simulink library "sps_library"  (R2025a)
settings: Solver=VariableStepAuto  StartTime=0.0  StopTime=10.0  RelTol=1e-3
undefined symbols (not defined in the file): bus, c_dc, gfli_b, inf_src, line_ns, ts
libraries: spsBreakerLib x7, spsabctodq0Lib x6, spsThreePhaseVIMeasurementLib x4, spsThreePhaseParallelRLCLoadLib x4, spsSeriesRLCBranchLib x3, spsThreePhaseSeriesRLCBranchLib x3, spsControlledCurrentSourceLib x2, spsDCVoltageSourceLib x2, spsGroundLib x2, spsThreePhaseBreakerLib x2, spsThreePhaseSourceLib x2, spsRMSLib x1
settings Model: Creator=paul  LastModifiedBy=paul

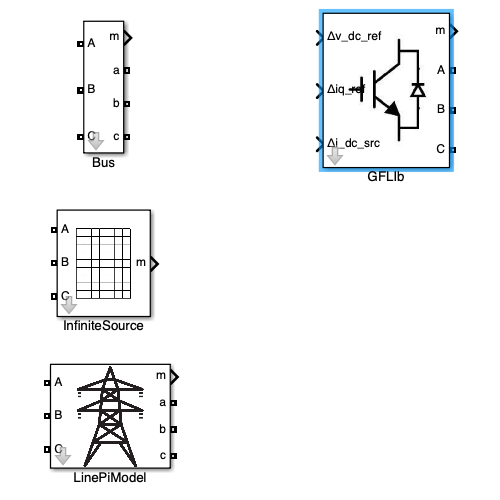
[thumbnail: Simulink's stored preview of the top-level diagram]
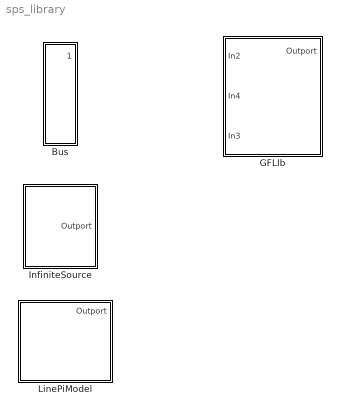
== system sps_library ==
  Bus : Subsystem  mask{s=bus{1}, sbase=100000000, vbase=230000, fbase=60}
      mask prompts: s "Structure from Workspace"; sbase "Sbase (3-phase VA)"; vbase "Vbase (L-L Vrms)"; fbase "Frequency (Hz)"
      mask init:
      | % Get simulink block as class. "m" is now a class
      | m = Simulink.Mask.get(gcb);
      | 
      | % Get an array of all parameters of the column "Name" of "Parameters & Dialog" tab
      | % For example, all_parameters = ['sbase', 'vbase']
      | all_parameters = m.Parameters;
      | 
      | % Iterate over all parameters and assign the field values of the structure
      | % in the workspace to the parameters of the current simulink block.
      | % The variable "st" must be defined in "Parameters & Dialog". 
      | 
      | for i = 1:numel(all_parameters)
      |     param_name = all_parameters(i).Name; % get parameter name of the simulink block
      |     if isfield(s, param_name) % check if field exist in the structure
      |         new_value = string(getfield(s, param_name)); % get the value of the structure field
      |         set_param(gcb, param_name, new_value); % assign the value of structure to simulink block
      |     end
      | end
      mask DialogControl DescGroupVar Prompt: Bus and measurements
      mask DialogControl Bus Prompt: Measure voltage, magnitude and phase, active power, reactive power. Note: Default current flow direction goes from uppercase (ABC) to lowercase (abc). Author: STING developers.
      mask DialogControl Container2 Prompt: Parameters
      mask DialogControl Control2 Prompt: Enter below the structure defined in your current Matlab workspace that contains parameters, power flow solution, initial conditions, etc. Click on "Apply" to migrate data to this block.
  GFLIb : Subsystem  mask{s=gfli_b{1}}
      mask prompts: s "Structure from workspace"
      mask init:
      | m = Simulink.Mask.get(gcb);
      |  
      | % Get all major boxes, like parameters, emt initial conditions
      | all_diagcontrols = m.getDialogControls();
      | 
      | for i=1:length(all_diagcontrols)
      | 
      |     control = all_diagcontrols(i);  
      |     control_name = control.Name; % name of box, for example: parameters, emt_init_cond
      |     control_fields = control.DialogControls; % all sub-boxes, like [sbase, vbase]
      | 
      |     for j=1:length(control_fields)
      | 
      |         param_name = control_fields(j).Name; % for example: sbase
      | 
      |         if isfield(s, param_name) % check if field exist in the structure
      |             new_value = string(getfield(s, param_name)); % get the value of the structure field
      |             set_param(gcb, param_name, new_value); % assign the value of structure to simulink block
      |         
      |         elseif isfield(s,control_name) % check if there is a structure inside of the structure
      |             x = getfield(s, control_name);
      |             if isfield(x, param_name)
      |                 new_value = string(getfield(x, param_name)); 
      |                 set_param(gcb, param_name, new_value);
      |             end
      | 
      |         end
      | 
      |     end
      | 
      | end
      mask DialogControl DescGroupVar Prompt: GFLIb
      mask DialogControl DescTextVar Prompt: Implements the GFLIb class from STING. It is a GFLI that includes PLL, L filter, current controller, and DC-side voltage controller. Author: STING developers.
      mask DialogControl Control2 Prompt: Enter below the structure defined in your current Matlab workspace that contains parameters, power flow solution, initial conditions, etc. Click on "Apply" to migrate data to this block.
      mask Display: image('IBR.jpeg');
  InfiniteSource : Subsystem  mask{s=inf_src{1}}
      mask prompts: s "Structure from workspace"
      mask init:
      | m = Simulink.Mask.get(gcb);
      | 
      | % Get all major boxes, like parameters, emt initial conditions
      | all_diagcontrols = m.getDialogControls();
      | 
      | for i=1:length(all_diagcontrols)
      | 
      |     control = all_diagcontrols(i);  
      |     control_name = control.Name; % name of box, for example: parameters, emt_init_cond
      |     control_fields = control.DialogControls; % all sub-boxes, like [sbase, vbase]
      | 
      |     for j=1:length(control_fields)
      | 
      |         param_name = control_fields(j).Name; % for example: sbase
      | 
      |         if isfield(s, param_name) % check if field exist in the structure
      |             new_value = string(getfield(s, param_name)); % get the value of the structure field
      |             set_param(gcb, param_name, new_value); % assign the value of structure to simulink block
      |         
      |         elseif isfield(s,control_name) % check if there is a structure inside of the structure
      |             x = getfield(s, control_name);
      |             new_value = string(getfield(x, param_name)); 
      |             set_param(gcb, param_name, new_value);
      | 
      |         end
      | 
      |     end
      | 
      | end
      mask DialogControl DescGroupVar Prompt: Infinite Source
      mask DialogControl DescTextVar Prompt: Implements the class InfiniteSource from STING. Author: STING developers.
      mask DialogControl Container2 Prompt: Parameters
      mask DialogControl Control2 Prompt: Enter below the structure defined in your current Matlab workspace that contains parameters, power flow solution, initial conditions, etc. Click on "Apply" to migrate data to this block.
      mask Display: image('grid.jpg', [0,0,0,0,80,80]);
  LinePiModel : Subsystem  mask{s=line_ns{1}}
      mask prompts: s "Structure from workspace"
      mask DialogControl DescGroupVar Prompt: Pi-model of transmission line
      mask DialogControl DescTextVar Prompt: Implements the class LinePiModel from STING. It is a transmission line that includes two shunt impendances and one series impendance. Author: STING developers.
      mask DialogControl Container2 Prompt: Parameters
      mask DialogControl Control2 Prompt: Enter below the structure defined in your current Matlab workspace that contains parameters, power flow solution, initial conditions, etc. Click on "Apply" to migrate data to this block.
      mask Display: image('tx_wo_se.jpg', [0,0,0,0,70,100]);

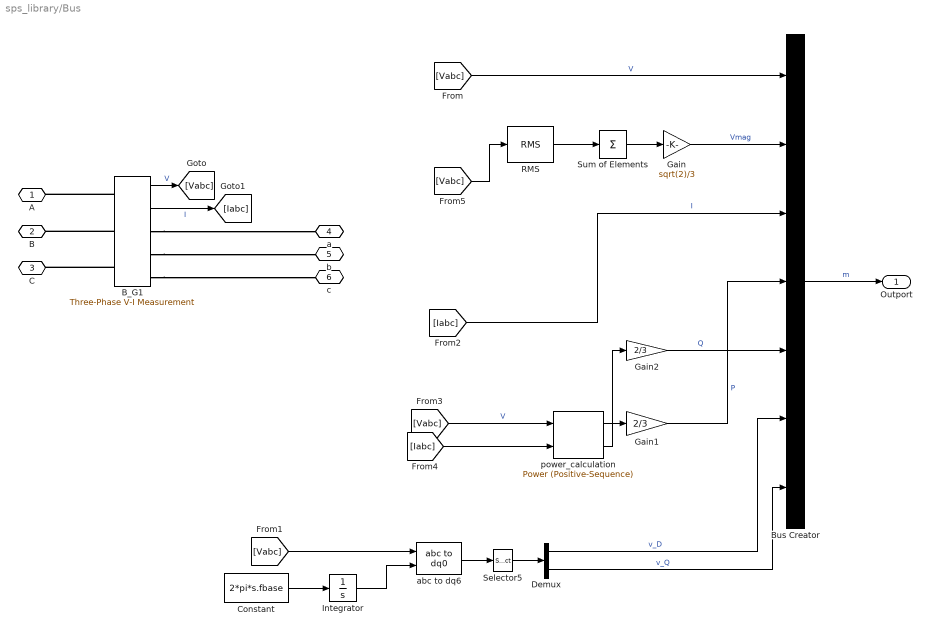
== system sps_library/Bus ==
  B_G1 : spsThreePhaseVIMeasurementLib/Three-Phase V-I Measurement  VoltageMeasurement=phase-to-ground  SetLabelV=off  LabelV=G1_Vabc  Vpu=on  VpuLL=off  CurrentMeasurement=yes  SetLabelI=off  LabelI=G1_Iabc  Ipu=on  Pbase=sbase  Vbase=vbase  OutputType=Complex  PhasorSimulation=off  PSBequivalent=0
  Bus Creator : BusCreator  Inputs=7
  Constant : Constant  Value=2*pi*s.fbase
  Demux : Demux  Outputs=2
  Gain : Gain  Gain=sqrt(2)/3
  Gain1 : Gain  Gain=2/3
  Gain2 : Gain  Gain=2/3
  Integrator : Integrator
  RMS : spsRMSLib/RMS  TrueRMS=on  Freq=fbase  RMSInit=1/sqrt(2)  Ts=0
  Selector5 : Selector  InputPortWidth=3  IndexOptions=Index vector (dialog)  Indices=[1 2]  OutputSizes=1
  Sum of Elements : Sum  Inputs=+
  abc to dq6 : spsabctodq0Lib/abc to dq0  Alignment=Aligned with phase A axis
  power_calculation : spsPowerPositiveSequenceLib/Power (Positive-Sequence)  Freq=fbase  Vinit=[1, 0]  Iinit=[0, 0]  Ts=ts
  A : PMIOPort  Side=Left
  B : PMIOPort  Port=2  Side=Left
  C : PMIOPort  Port=3  Side=Left
  a : PMIOPort  Port=4  Side=Right
  b : PMIOPort  Port=5  Side=Right
  c : PMIOPort  Port=6  Side=Right
  Outport : Outport
  wires:
  Bus Creator/1 -> Outport/1  "m"
  Gain1/1 -> Bus Creator/4  "P"
  Gain2/1 -> Bus Creator/5  "Q"
  B_G1/1 -> [Vabc]  "V"
  [Vabc] -> Bus Creator/1  "V"
  B_G1/2 -> [Iabc]  "I"
  [Iabc] -> Bus Creator/3  "I"
  [Vabc] -> power_calculation/1  "V"
  [Vabc] -> RMS/1
  RMS/1 -> Sum of Elements/1
  Sum of Elements/1 -> Gain/1
  Gain/1 -> Bus Creator/2  "Vmag"
  power_calculation/1 -> Gain1/1
  [Iabc] -> power_calculation/2
  power_calculation/2 -> Gain2/1
  [Vabc] -> abc to dq6/1
  Demux/2 -> Bus Creator/7  "v_Q"
  Integrator/1 -> abc to dq6/2
  Selector5/1 -> Demux/1
  Constant/1 -> Integrator/1
  Demux/1 -> Bus Creator/6  "v_D"
  abc to dq6/1 -> Selector5/1
  connections:
  B_G1/LConn1 -- A/RConn1
  B_G1/LConn3 -- C/RConn1
  B_G1/RConn2 -- b/RConn1
  B_G1/RConn1 -- a/RConn1
  B_G1/LConn2 -- B/RConn1
  B_G1/RConn3 -- c/RConn1

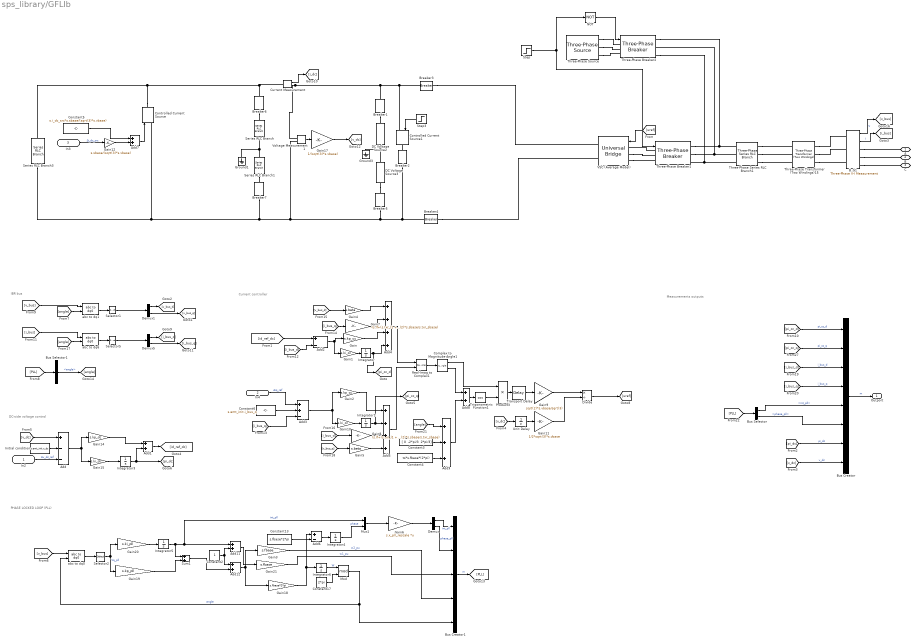
== system sps_library/GFLIb ==
  note: IBR bus
  note: Current controller
  note: Measurements outputs
  note: PHASE LOCKED LOOP (PLL)
  note: DC-side voltage control
  In2 : Inport
  In4 : Inport  Port=2
  In3 : Inport  Port=3
  Add : Sum  Inputs=+--
  Add{1,7..8,11..12} (5 alike) : Sum
  Add2 : Sum  Inputs=+-
  Add3 : Sum  Inputs=++-
  Add4 : Sum  Inputs=++++
  Add5 : Sum  Inputs=++++
  Add6 : Sum  Inputs=+-
  Add9 : Sum  Inputs=+++
  B_G1 : spsThreePhaseVIMeasurementLib/Three-Phase V-I Measurement  VoltageMeasurement=phase-to-ground  SetLabelV=off  LabelV=G1_Vabc  Vpu=on  VpuLL=off  CurrentMeasurement=yes  SetLabelI=off  LabelI=G1_Iabc  Ipu=on  Pbase=s.sbase  Vbase=230*10^3  OutputType=Complex  PhasorSimulation=off  PSBequivalent=0
  Breaker1 : spsBreakerLib/Breaker  InitialState=1  SwitchingTimes=[ts]  External=off  BreakerResistance=1e-7  SnubberResistance=1e6  SnubberCapacitance=inf  Measurements=None  MoreParameters=on  NoBreakLoop=off
  Breaker2 : spsBreakerLib/Breaker  InitialState=1  SwitchingTimes=[ts]  External=off  BreakerResistance=1e-7  SnubberResistance=1e6  SnubberCapacitance=inf  Measurements=None  MoreParameters=on  NoBreakLoop=off
  Breaker{3..4,6..7} (4 alike) : spsBreakerLib/Breaker  InitialState=0  SwitchingTimes=[ts]  External=off  BreakerResistance=1e-7  SnubberResistance=1e6  SnubberCapacitance=inf  Measurements=None  MoreParameters=on  NoBreakLoop=off
  Breaker5 : spsBreakerLib/Breaker  InitialState=1  SwitchingTimes=[ts]  External=off  BreakerResistance=1e-7  SnubberResistance=1e6  SnubberCapacitance=inf  Measurements=None  MoreParameters=on  NoBreakLoop=off
  Bus Creator : BusCreator  Inputs=8
  Bus Creator1 : BusCreator  Inputs=5
  Bus Selector : BusSelector  OutputSignals=int_pll,phase_pll
  Bus Selector1 : BusSelector  OutputSignals=angle
  Complex to Magnitude-Angle1 : ComplexToMagnitudeAngle
  Constant13 : Constant  Value=s.fbase*2*pi
  Constant17 : Constant  Value=2*pi
  Constant2 : Constant
  Constant3 : Constant  Value="[ 0  -2*pi/3  2*pi/3]"
  Constant4 : Constant  Value=ts*s.fbase*(2*pi)
  Constant5 : Constant  Value=s.i_dc_src*s.sbase/(sqrt(3)*s.vbase)
  Constant6 : Constant  Value=s.emt_init.i_bus_q
  Controlled Current Source : spsControlledCurrentSourceLib/Controlled Current Source  Initialize=off  Source_Type=AC  Amplitude=0  Phase=0  Frequency=0  Measurements=None
  Controlled Current Source1 : spsControlledCurrentSourceLib/Controlled Current Source  Initialize=off  Source_Type=AC  Amplitude=0  Phase=0  Frequency=0  Measurements=None
  Current Measurement : spsCurrentMeasurementLib/Current Measurement  PhasorSimulation=off  OutputType=Complex  PSBequivalent=0
  DC Voltage Source2 : spsDCVoltageSourceLib/DC Voltage Source  Amplitude=+sqrt(3)*s.vbase*s.emt_init.v_dc/2  Measurements=None
  DC Voltage Source3 : spsDCVoltageSourceLib/DC Voltage Source  Amplitude=+sqrt(3)*s.vbase*s.emt_init.v_dc/2  Measurements=None
  Demux : Demux  Outputs=2
  Demux1 : Demux  Outputs=2
  Demux5 : Demux  Outputs=2
  Divide : Product  Inputs=*/
  Gain : Gain  Gain=s.kp_cc
  Gain1 : Gain  Gain=s.ki_cc
  Gain10 : Gain  Gain=s.ki_cc
  Gain11 : Gain  Gain=1/2*sqrt(3)*s.vbase
  Gain12 : Gain  Gain=s.sbase/(sqrt(3)*s.vbase)
  Gain14 : Gain  Gain=s.kp_dc
  Gain15 : Gain  Gain=s.ki_dc
  Gain17 : Gain  Gain=1/(sqrt(3)*s.vbase)
  Gain18 : Gain  Gain=s.fbase*2*pi
  Gain19 : Gain  Gain=s.kp_pll
  Gain2 : Gain  Gain=s.kp_cc
  Gain20 : Gain  Gain=s.ki_pll
  Gain21 : Gain  Gain=s.fbase
  Gain3 : Gain  Gain=s.fbase
  Gain4 : Gain  Gain=s.beta
  Gain5 : Gain  Gain=s.beta
  Gain6 : Gain  Gain=s.x_pll_rescale  Multiplication=Matrix(K*u)
  Gain7 : Gain  Gain=-(s.lf+(s.txr_l1 + s.txr_l2)*s.sbase/s.txr_sbase)
  Gain8 : Gain  Gain=(s.lf+(s.txr_l1 + s.txr_l2)*s.sbase/s.txr_sbase)
  Gain9 : Gain  Gain=sqrt(2)*s.vbase/sqrt(3)
  Ground1 : spsGroundLib/Ground  LConnTagsString=a
  Ground3 : spsGroundLib/Ground  LConnTagsString=a
  Initial condition : Constant  Value=s.emt_init.v_dc
  Integrator : Integrator  InitialCondition=s.emt_init.pi_cc_d
  Integrator1 : Integrator  InitialCondition=s.emt_init.pi_cc_q
  Integrator3 : Integrator  InitialCondition=s.emt_init.i_bus_d
  Integrator4 : Integrator  InitialCondition=s.emt_init.angle_ref*pi/180
  Integrator5 : Integrator
  Integrator6 : Integrator  InitialCondition=s.emt_init.angle_ref*pi/180
  Mod : Math  Operator=mod
  Mux1 : Mux  Inputs=2
  NOT : Logic  Operator=NOT  IconShape=distinctive  AllPortsSameDT=off  OutDataTypeStr=boolean
  Product3 : Product  Inputs=**  RndMeth=Zero
  Real-Imag to Complex1 : RealImagToComplex
  Selector1 : Selector  InputPortWidth=3  IndexOptions=Index vector (dialog)  Indices=[1 2]  OutputSizes=1
  Selector2 : Selector  InputPortWidth=3  IndexOptions=Index vector (dialog)  Indices=2  OutputSizes=1
  Selector5 : Selector  InputPortWidth=3  IndexOptions=Index vector (dialog)  Indices=[1 2]  OutputSizes=1
  Series RLC Branch : spsSeriesRLCBranchLib/Series RLC Branch  LConnTagsString=__new0  RConnTagsString=__new0  BranchType=C  Resistance=1  Inductance=1e-3  SetiL0=off  InitialCurrent=0  Capacitance=s.c_dc*1/(3*s.vbase^2/s.sbase)*1/(2*pi*s.fbase)  Setx0=on  InitialVoltage=+sqrt(3)*s.vbase*s.emt_init.v_dc/2  Measurements=None
  Series RLC Branch1 : spsSeriesRLCBranchLib/Series RLC Branch  LConnTagsString=__new0  RConnTagsString=__new0  BranchType=C  Resistance=1  Inductance=1e-3  SetiL0=off  InitialCurrent=0  Capacitance=s.c_dc*1/(3*s.vbase^2/s.sbase)*1/(2*pi*s.fbase)  Setx0=on  InitialVoltage=+sqrt(3)*s.vbase*s.emt_init.v_dc/2  Measurements=None
  Series RLC Branch3 : spsSeriesRLCBranchLib/Series RLC Branch  LConnTagsString=__new0  RConnTagsString=__new0  BranchType=R  Resistance=s.r_dc*(3*s.vbase^2/s.sbase)  Inductance=1e-3  SetiL0=off  InitialCurrent=0  Capacitance=c_dc  Setx0=off  InitialVoltage=0  Measurements=None
  Step : Step  Time=ts  SampleTime=0
  Step3 : Step  Time=ts  Before=s.emt_init.i_out*s.sbase/(sqrt(3)*s.vbase)  After=0  SampleTime=ts
  Sum1 : Sum  SaturateOnIntegerOverflow=on
  Three-Phase Series RLC Branch1 : spsThreePhaseSeriesRLCBranchLib/Three-Phase Series RLC Branch  LConnTagsString=A|B|C  RConnTagsString=A|B|C  BranchType=RL  Resistance=s.rf * s.vbase^2/s.sbase  Inductance=s.lf * s.vbase^2/s.sbase * 1/(2*pi*s.fbase)  Capacitance=1e-6  Measurements=None
  Three-Phase Transformer (Two Windings)15 : spsThreePhaseTransformerTwoWindingsLib/Three-Phase Transformer (Two Windings)  Winding1Connection=Yg  Winding2Connection=Yg  CoreType=Three single-phase transformers  SetSaturation=off  Hysteresis=off  DataFile='hysteresis'  SetInitialFlux=off  Measurements=None  UNITS=pu  NominalPower=[s.txr_sbase , s.fbase ]  Winding1=[ s.vbase , s.txr_r1 , s.txr_l1 ]  Winding2=[ 230*10^3 , s.txr_r2 , s.txr_l2 ]  Rm=1000  Lm=inf  L0=2.866  Saturation=[ 0,0 ; 0.0024,1.2 ; 1.0,1.52 ]  InitialFluxes=[1273.5 -1273.5 1114.3]  BreakLoop=off  DiscreteSolver=Trapezoidal robust  DataType=off  TransfoNumber=1
  Three-Phase Breaker1 : spsThreePhaseBreakerLib/Three-Phase Breaker  InitialState=open  SwitchA=on  SwitchB=on  SwitchC=on  SwitchTimes="[1/60  5/60]"  External=on  BreakerResistance=1e-7  SnubberResistance=1e6  SnubberCapacitance=inf  Measurements=None
  Three-Phase Breaker2 : spsThreePhaseBreakerLib/Three-Phase Breaker  InitialState=closed  SwitchA=on  SwitchB=on  SwitchC=on  SwitchTimes="[1/60  5/60]"  External=on  BreakerResistance=1e-7  SnubberResistance=1e6  SnubberCapacitance=inf  Measurements=None
  Three-Phase Source : spsThreePhaseSourceLib/Three-Phase Source  InternalConnection=Yg  VoltagePhases=off  Voltage=s.emt_init.v_vsc_mag*s.vbase  PhaseAngle=90+s.emt_init.v_vsc_DQ_phase  Voltage_phases=[25e3 25e3 25e3]/sqrt(3)  PhaseAngles_phases=[0 -120 +120]  Frequency=s.fbase  NonIdealSource=off  SpecifyImpedance=off  Resistance=0.8929  Inductance=16.58e-3  ShortCircuitLevel=100e6  BaseVoltage=25e3  XRratio=7  BusType=swing  Pref=10e3  Qref=0  Prefabc=[10e3, 10e3, 10e3]  Qrefabc=[0, 0, 0]  Qmin=-inf  Qmax=inf
  Transport Delay : TransportDelay  DelayTime=ts  InitialOutput=s.emt_init.v_vsc_mag*[cosd(s.emt_init.v_vsc_DQ_phase) cosd(s.emt_init.v_vsc_DQ_phase-120) cosd(s.emt_init.v_vsc_DQ_phase+120)]
  Trigonometric Function1 : Trigonometry  Operator=cos
  Unit Delay : UnitDelay  InitialCondition=s.emt_init.v_dc  SampleTime=ts  HasFrameUpgradeWarning=on
  VSC (Average Model) : spsUniversalBridgeLib/Universal Bridge  Arms=3  SnubberResistance=1e5  SnubberCapacitance=inf  Device=Average-model based VSC  Ron=1e-3  Lon=0  ForwardVoltages="[  0  0  ]"  ForwardVoltage=0  GTOparameters=[ 10e-6 , 20e-6 ]  IGBTparameters=[ 1e-6 , 2e-6 ]  Measurements=None  Measurements_2=None  converterType=Rectifier
  Voltage Measurement1 : spsVoltageMeasurementLib/Voltage Measurement  PhasorSimulation=off  OutputType=Complex  PSBequivalent=0
  abc to dq0 : spsabctodq0Lib/abc to dq0  Alignment=Aligned with phase A axis
  abc to dq1 : spsabctodq0Lib/abc to dq0  Alignment=Aligned with phase A axis
  abc to dq6 : spsabctodq0Lib/abc to dq0  Alignment=Aligned with phase A axis
  A : PMIOPort  Side=Right
  B : PMIOPort  Port=2  Side=Right
  C : PMIOPort  Port=3  Side=Right
  Outport : Outport
  wires:
  Add8/1 -> Trigonometric Function1/1
  [uref] -> VSC (Average Model)/1
  Add5/1 -> Real-Imag to Complex1/2
  Constant3/1 -> Add9/2
  Gain7/1 -> Add4/2
  Gain9/1 -> Divide/1
  Trigonometric Function1/1 -> Product3/2
  [angle] -> Add9/1
  Complex to Magnitude-Angle1/2 -> Add8/1
  Add2/1 -> Gain1/1, Gain/1
  Demux5/2 -> [i_bus_q]
  [angle] -> abc to dq6/2
  Gain4/1 -> Add4/1
  [v_bus_q] -> Gain5/1
  Product3/1 -> Transport Delay/1
  [i_bus] -> abc to dq6/1
  [v_bus_d] -> Gain4/1
  Add4/1 -> Real-Imag to Complex1/1
  Real-Imag to Complex1/1 -> Complex to Magnitude-Angle1/1
  [i_bus_q] -> Gain7/1
  Complex to Magnitude-Angle1/1 -> Product3/1
  abc to dq6/1 -> Selector5/1
  Add9/1 -> Add8/2
  Constant4/1 -> Add9/3
  [i_bus_d] -> Gain8/1
  Gain/1 -> Add4/3
  Demux5/1 -> [i_bus_d]
  Integrator/1 -> Add4/4, [pi_cc_d]
  Gain5/1 -> Add5/4
  Gain8/1 -> Add5/3
  Gain2/1 -> Add5/1
  Add3/1 -> Gain10/1, Gain2/1
  abc to dq1/1 -> Selector1/1
  Demux1/1 -> [v_bus_d]
  Demux1/2 -> [v_bus_q]
  [v_bus] -> abc to dq1/1
  [angle] -> abc to dq1/2
  Gain1/1 -> Integrator/1
  Integrator1/1 -> [pi_cc_q], Add5/2
  Gain10/1 -> Integrator1/1
  Selector1/1 -> Demux1/1
  Selector5/1 -> Demux5/1
  NOT/1 -> Three-Phase Breaker2/1
  Step/1 -> NOT/1, Three-Phase Breaker1/1
  Transport Delay/1 -> Gain9/1
  In4/1 -> Add3/1  "Δiq_ref"
  [pi_cc_d] -> Bus Creator/1  "pi_cc_d"
  [pi_cc_q] -> Bus Creator/2  "pi_cc_q"
  Bus Creator/1 -> Outport/1  "m"
  [i_bus_d] -> Bus Creator/3  "i_bus_d"
  [i_bus_q] -> Bus Creator/4  "i_bus_q"
  [v_dc] -> Unit Delay/1
  Gain11/1 -> Divide/2
  Divide/1 -> [uref]
  B_G1/1 -> [v_bus]  "V"
  B_G1/2 -> [i_bus]  "I"
  [i_bus_q] -> Add3/3
  Constant6/1 -> Add3/2
  Unit Delay/1 -> Gain11/1
  [i_bus_d] -> Add2/2
  In3/1 -> Gain12/1  "Δi_dc_src"
  Voltage Measurement1/1 -> Gain17/1
  Current Measurement/1 -> [i_dc]
  Step3/1 -> Controlled Current Source1/1
  Add7/1 -> Controlled Current Source/1
  Gain17/1 -> [v_dc]
  Constant5/1 -> Add7/1
  Integrator3/1 -> [pi_dc], Add1/2
  Add1/1 -> [id_ref_dc]
  Gain15/1 -> Integrator3/1
  [v_dc] -> Add/1
  Initial condition/1 -> Add/2
  Add/1 -> Gain15/1, Gain14/1
  In2/1 -> Add/3  "Δv_dc_ref"
  Gain14/1 -> Add1/1
  [pi_dc] -> Bus Creator/7  "pi_dc"
  [v_dc] -> Bus Creator/8  "v_dc"
  [id_ref_dc] -> Add2/1
  Constant13/1 -> Add6/2
  Selector2/1 -> Gain20/1, Gain19/1  "Vq_pll"
  Constant17/1 -> Mod/2
  Bus Creator1/1 -> [PLL]  "m"
  Constant2/1 -> Add12/1, Add11/2
  Integrator4/1 -> Mux1/2  "phase"
  Add11/1 -> Gain21/1
  Add12/1 -> Gain18/1, Gain3/1
  Integrator6/1 -> Mod/1  "W"
  Mod/1 -> abc to dq0/2, Bus Creator1/5  "angle"
  Gain18/1 -> Integrator6/1, Add6/1
  Gain20/1 -> Integrator5/1
  Gain3/1 -> Bus Creator1/4  "w2_pu"
  [v_bus] -> abc to dq0/1
  Sum1/1 -> Add12/2
  abc to dq0/1 -> Selector2/1
  Gain19/1 -> Sum1/2
  Add6/1 -> Integrator4/1
  Gain21/1 -> Bus Creator1/3  "w1_pu"
  Bus Selector1/1 -> [angle]  "<angle>"
  [PLL] -> Bus Selector1/1
  [PLL] -> Bus Selector/1
  Integrator5/1 -> Mux1/1, Add11/1, Sum1/1  "int_pll"
  Bus Selector/1 -> Bus Creator/5  "<int_pll>"
  Bus Selector/2 -> Bus Creator/6  "<phase_pll>"
  Mux1/1 -> Gain6/1
  Gain6/1 -> Demux/1
  Demux/1 -> Bus Creator1/1  "int_pll"
  Demux/2 -> Bus Creator1/2  "phase_pll"
  Gain12/1 -> Add7/2
  connections:
  Three-Phase Source/RConn3 -- Three-Phase Breaker2/LConn3
  Three-Phase Source/RConn2 -- Three-Phase Breaker2/LConn2
  Three-Phase Source/RConn1 -- Three-Phase Breaker2/LConn1
  Three-Phase Breaker1/LConn1 -- VSC (Average Model)/LConn1
  VSC (Average Model)/LConn2 -- Three-Phase Breaker1/LConn2
  VSC (Average Model)/LConn3 -- Three-Phase Breaker1/LConn3
  Three-Phase Breaker1/RConn2 -- Three-Phase Series RLC Branch1/LConn2 -- Three-Phase Breaker2/RConn2
  Three-Phase Breaker1/RConn1 -- Three-Phase Breaker2/RConn1 -- Three-Phase Series RLC Branch1/LConn1
  B_G1/RConn1 -- A/RConn1
  B_G1/RConn2 -- B/RConn1
  B_G1/RConn3 -- C/RConn1
  Three-Phase Breaker2/RConn3 -- Three-Phase Breaker1/RConn3 -- Three-Phase Series RLC Branch1/LConn3
  Three-Phase Series RLC Branch1/RConn1 -- Three-Phase Transformer (Two Windings)15/LConn1
  Three-Phase Series RLC Branch1/RConn2 -- Three-Phase Transformer (Two Windings)15/LConn2
  Three-Phase Series RLC Branch1/RConn3 -- Three-Phase Transformer (Two Windings)15/LConn3
  Three-Phase Transformer (Two Windings)15/RConn1 -- B_G1/LConn1
  Three-Phase Transformer (Two Windings)15/RConn2 -- B_G1/LConn2
  Three-Phase Transformer (Two Windings)15/RConn3 -- B_G1/LConn3
  Controlled Current Source/LConn1 -- Series RLC Branch3/RConn1 -- Voltage Measurement1/LConn2 -- Breaker4/RConn1 -- Breaker2/RConn1 -- Breaker5/RConn1 -- Breaker7/RConn1
  Voltage Measurement1/LConn1 -- Current Measurement/RConn1 -- Breaker1/LConn1 -- Breaker3/RConn1 -- Controlled Current Source1/LConn1
  Controlled Current Source/RConn1 -- Series RLC Branch3/LConn1 -- Breaker6/LConn1 -- Current Measurement/LConn1
  DC Voltage Source2/LConn1 -- DC Voltage Source3/RConn1 -- Ground3/LConn1
  Series RLC Branch/RConn1 -- Series RLC Branch1/LConn1 -- Ground1/LConn1
  Breaker4/LConn1 -- VSC (Average Model)/RConn2
  Breaker2/LConn1 -- Controlled Current Source1/RConn1
  Breaker6/RConn1 -- Series RLC Branch/LConn1
  Breaker1/RConn1 -- DC Voltage Source2/RConn1
  Breaker3/LConn1 -- VSC (Average Model)/RConn1
  DC Voltage Source3/LConn1 -- Breaker5/LConn1
  Series RLC Branch1/RConn1 -- Breaker7/LConn1

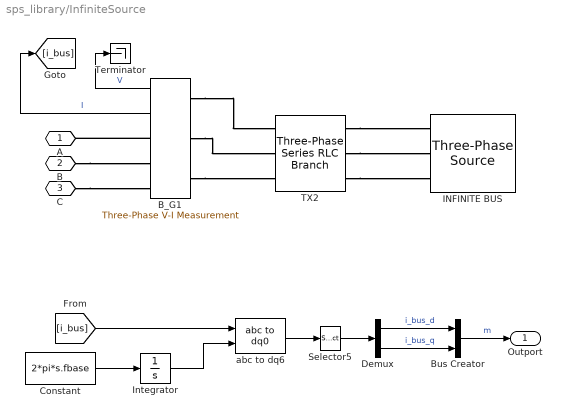
== system sps_library/InfiniteSource ==
  B_G1 : spsThreePhaseVIMeasurementLib/Three-Phase V-I Measurement  VoltageMeasurement=phase-to-ground  SetLabelV=off  LabelV=G1_Vabc  Vpu=on  VpuLL=off  CurrentMeasurement=yes  SetLabelI=off  LabelI=G1_Iabc  Ipu=on  Pbase=s.sbase  Vbase=s.vbase  OutputType=Complex  PhasorSimulation=off  PSBequivalent=0
  Bus Creator : BusCreator  Inputs=2
  Constant : Constant  Value=2*pi*s.fbase
  Demux : Demux  Outputs=2
  INFINITE BUS : spsThreePhaseSourceLib/Three-Phase Source  InternalConnection=Yg  VoltagePhases=off  Voltage=s.vbase*s.emt_init.v_int_d  PhaseAngle=90+s.emt_init.angle_ref  Voltage_phases=[25e3 25e3 25e3]/sqrt(3)  PhaseAngles_phases=[0 -120 +120]  Frequency=s.fbase  NonIdealSource=off  SpecifyImpedance=off  Resistance=0.8929  Inductance=16.58e-3  ShortCircuitLevel=100e6  BaseVoltage=SYSPAR.vbase  XRratio=7  BusType=swing  Pref=10000  Qref=0  Prefabc=[10e3, 10e3, 10e3]  Qrefabc=[0, 0, 0]  Qmin=-Inf  Qmax=Inf
  Integrator : Integrator  InitialCondition=s.emt_init.angle_ref*pi/180
  Selector5 : Selector  InputPortWidth=3  IndexOptions=Index vector (dialog)  Indices=[1 2]  OutputSizes=1
  TX2 : spsThreePhaseSeriesRLCBranchLib/Three-Phase Series RLC Branch  LConnTagsString=A|B|C  RConnTagsString=A|B|C  BranchType=RL  Resistance=s.r*s.vbase^2/s.sbase  Inductance=s.l*s.vbase^2/s.sbase*1/(2*pi*s.fbase)  Capacitance=0.00961998 / 120 / pi  Measurements=Branch voltages
  Terminator : Terminator
  abc to dq6 : spsabctodq0Lib/abc to dq0  Alignment=Aligned with phase A axis
  A : PMIOPort  Side=Left
  B : PMIOPort  Port=2  Side=Left
  C : PMIOPort  Port=3  Side=Left
  Outport : Outport
  wires:
  abc to dq6/1 -> Selector5/1
  B_G1/2 -> [i_bus]  "I"
  B_G1/1 -> Terminator/1  "V"
  [i_bus] -> abc to dq6/1
  Constant/1 -> Integrator/1
  Integrator/1 -> abc to dq6/2
  Selector5/1 -> Demux/1
  Demux/1 -> Bus Creator/1  "i_bus_d"
  Demux/2 -> Bus Creator/2  "i_bus_q"
  Bus Creator/1 -> Outport/1  "m"
  connections:
  TX2/RConn2 -- INFINITE BUS/RConn2
  TX2/RConn1 -- INFINITE BUS/RConn1
  TX2/RConn3 -- INFINITE BUS/RConn3
  B_G1/LConn1 -- TX2/LConn1
  B_G1/LConn2 -- TX2/LConn2
  B_G1/LConn3 -- TX2/LConn3
  B_G1/RConn1 -- A/RConn1
  B/RConn1 -- B_G1/RConn2
  C/RConn1 -- B_G1/RConn3

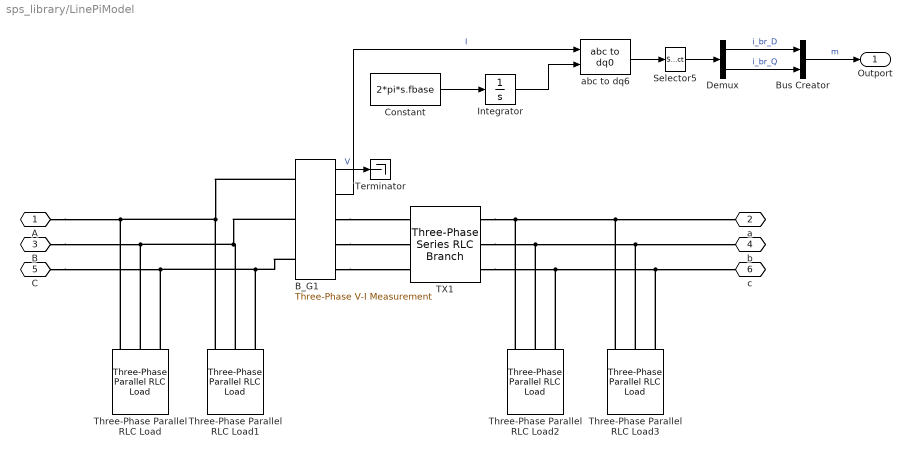
== system sps_library/LinePiModel ==
  B_G1 : spsThreePhaseVIMeasurementLib/Three-Phase V-I Measurement  VoltageMeasurement=phase-to-ground  SetLabelV=off  LabelV=G1_Vabc  Vpu=on  VpuLL=off  CurrentMeasurement=yes  SetLabelI=off  LabelI=G1_Iabc  Ipu=on  Pbase=s.sbase  Vbase=s.vbase  OutputType=Complex  PhasorSimulation=off  PSBequivalent=0
  Bus Creator : BusCreator  Inputs=2
  Constant : Constant  Value=2*pi*s.fbase
  Demux : Demux  Outputs=2
  Integrator : Integrator
  Selector5 : Selector  InputPortWidth=3  IndexOptions=Index vector (dialog)  Indices=[1 2]  OutputSizes=1
  TX1 : spsThreePhaseSeriesRLCBranchLib/Three-Phase Series RLC Branch  LConnTagsString=A|B|C  RConnTagsString=A|B|C  BranchType=RL  Resistance=s.r *s.vbase^2/s.sbase  Inductance=s.l * s.vbase^2/s.sbase*1/(2*pi*s.fbase)  Capacitance=0.00961998 / 120 / pi  Measurements=Branch voltages
  Terminator : Terminator
  Three-Phase Parallel RLC Load : spsThreePhaseParallelRLCLoadLib/Three-Phase Parallel RLC Load  LConnTagsString=A|B|C  Configuration=Y (grounded)  NominalVoltage=s.vbase  Vabc=[1e3 1e3 1e3]  Vabcp=[1e3 1e3 1e3]  NominalFrequency=s.fbase  UnbalancedPower=off  ActivePower=s.g*s.sbase  InductivePower=0  CapacitivePower=0  Pabc=[10e3 9e3 11e3]  QLabc=[100 90 110]  QCabc=[100 90 110]  Pabcp=[10e3 9e3 11e3]  QLabcp=[100 90 110]  QCabcp=[100 90 110]  Measurements=None  LoadType=constant Z
  Three-Phase Parallel RLC Load1 : spsThreePhaseParallelRLCLoadLib/Three-Phase Parallel RLC Load  LConnTagsString=A|B|C  Configuration=Y (grounded)  NominalVoltage=s.vbase  Vabc=[1e3 1e3 1e3]  Vabcp=[1e3 1e3 1e3]  NominalFrequency=s.fbase  UnbalancedPower=off  ActivePower=0  InductivePower=0  CapacitivePower=s.b*s.sbase  Pabc=[10e3 9e3 11e3]  QLabc=[100 90 110]  QCabc=[100 90 110]  Pabcp=[10e3 9e3 11e3]  QLabcp=[100 90 110]  QCabcp=[100 90 110]  Measurements=None  LoadType=constant Z
  Three-Phase Parallel RLC Load2 : spsThreePhaseParallelRLCLoadLib/Three-Phase Parallel RLC Load  LConnTagsString=A|B|C  Configuration=Y (grounded)  NominalVoltage=s.vbase  Vabc=[1e3 1e3 1e3]  Vabcp=[1e3 1e3 1e3]  NominalFrequency=s.fbase  UnbalancedPower=off  ActivePower=s.g*s.sbase  InductivePower=0  CapacitivePower=0  Pabc=[10e3 9e3 11e3]  QLabc=[100 90 110]  QCabc=[100 90 110]  Pabcp=[10e3 9e3 11e3]  QLabcp=[100 90 110]  QCabcp=[100 90 110]  Measurements=None  LoadType=constant Z
  Three-Phase Parallel RLC Load3 : spsThreePhaseParallelRLCLoadLib/Three-Phase Parallel RLC Load  LConnTagsString=A|B|C  Configuration=Y (grounded)  NominalVoltage=s.vbase  Vabc=[1e3 1e3 1e3]  Vabcp=[1e3 1e3 1e3]  NominalFrequency=s.fbase  UnbalancedPower=off  ActivePower=0  InductivePower=0  CapacitivePower=s.b*s.sbase  Pabc=[10e3 9e3 11e3]  QLabc=[100 90 110]  QCabc=[100 90 110]  Pabcp=[10e3 9e3 11e3]  QLabcp=[100 90 110]  QCabcp=[100 90 110]  Measurements=None  LoadType=constant Z
  abc to dq6 : spsabctodq0Lib/abc to dq0  Alignment=Aligned with phase A axis
  A : PMIOPort  Side=Left
  a : PMIOPort  Port=2  Side=Right
  B : PMIOPort  Port=3  Side=Left
  b : PMIOPort  Port=4  Side=Right
  C : PMIOPort  Port=5  Side=Left
  c : PMIOPort  Port=6  Side=Right
  Outport : Outport
  wires:
  B_G1/1 -> Terminator/1  "V"
  Demux/1 -> Bus Creator/1  "i_br_D"
  abc to dq6/1 -> Selector5/1
  Selector5/1 -> Demux/1
  Demux/2 -> Bus Creator/2  "i_br_Q"
  Integrator/1 -> abc to dq6/2
  Constant/1 -> Integrator/1
  B_G1/2 -> abc to dq6/1  "I"
  Bus Creator/1 -> Outport/1  "m"
  connections:
  TX1/RConn1 -- Three-Phase Parallel RLC Load2/LConn1 -- Three-Phase Parallel RLC Load3/LConn1 -- a/RConn1
  TX1/RConn3 -- Three-Phase Parallel RLC Load3/LConn3 -- c/RConn1 -- Three-Phase Parallel RLC Load2/LConn3
  TX1/RConn2 -- Three-Phase Parallel RLC Load2/LConn2 -- Three-Phase Parallel RLC Load3/LConn2 -- b/RConn1
  A/RConn1 -- Three-Phase Parallel RLC Load1/LConn1 -- B_G1/LConn1 -- Three-Phase Parallel RLC Load/LConn1
  B/RConn1 -- B_G1/LConn2 -- Three-Phase Parallel RLC Load1/LConn2 -- Three-Phase Parallel RLC Load/LConn2
  C/RConn1 -- B_G1/LConn3 -- Three-Phase Parallel RLC Load1/LConn3 -- Three-Phase Parallel RLC Load/LConn3
  B_G1/RConn1 -- TX1/LConn1
  B_G1/RConn2 -- TX1/LConn2
  B_G1/RConn3 -- TX1/LConn3
